simulink model "simulator_prototype_v2"  (R2021b)
settings: Solver=VariableStepAuto  StartTime=0.0  StopTime=60  FixedStep=0.0001  RelTol=1e-4
undefined symbols (not defined in the file or in its folder): X, Y, Z
libraries: sm_lib x47, nesl_utility x7
(part 13 of 13)

== matlab function simulator_prototype_v2/Energy Analysis/MATLAB Function ==
  data: dq input; T output; H input
function T = Kinetic_Energy(dq, H)
T = real((1/2)*transpose(dq)*H*dq);

== matlab function simulator_prototype_v2/Energy Analysis/potential_energy ==
  data: q1 input; U output; q2 input; q3 input; q4 input; q5 input; q6 input
function U = potential_energy(q1,q2,q3,q4,q5,q6)
%#codegen

%    This function was generated by the Symbolic Math Toolbox version 9.0.
%    12-Oct-2021 13:17:17

t2 = conj(q1);
t3 = conj(q2);
t4 = conj(q3);
t5 = conj(q4);
t6 = conj(q5);
t7 = conj(q6);
t24 = 9.007199254740992e+15;
t8 = cos(t2);
t9 = cos(t3);
t10 = cos(t5);
t11 = cos(t6);
t12 = cos(t7);
t13 = sin(t2);
t14 = sin(t3);
t15 = sin(t5);
t16 = sin(t6);
t17 = sin(t7);
t18 = t2+t3;
t26 = (t4.*t24)./9.007199254740992e+15;
t29 = t4.*t24.*1.110223024625157e-16i;
t19 = cos(t18);
t20 = sin(t18);
t27 = cos(t26);
t28 = sin(t26);
t30 = -t29;
t31 = exp(t29);
t21 = t20.*4.602992943936994e+15;
t22 = t19.*7.742227997977903e+15;
t32 = -t27;
t33 = exp(t30);
t34 = t28.*1i;
t38 = t27.*7.38843356682345e-1;
t39 = t27.*2.61156643317655e-1;
t23 = -t21;
t35 = t33-1.0;
t37 = t27+t34;
t40 = t32+t34+1.0;
t42 = t10.*t24.*t28.*(t21-t22).*(-1.232595164407831e-32);
t43 = t15.*t24.*t28.*(t21-t22).*(-1.232595164407831e-32);
t44 = (t10.*t24.*t28.*(t21-t22))./8.112963841460668e+31;
t45 = t38+2.61156643317655e-1;
t46 = t39+7.38843356682345e-1;
t25 = t22+t23;
t36 = t35.^2;
t41 = t40.^2;
t47 = t19.*t45;
t48 = t20.*t46;
t49 = t20.*t37.*t41.*2.196325630278387e-1;
t50 = t19.*t37.*t41.*2.196325630278387e-1;
t51 = -t49;
t52 = -t50;
t53 = t47+t51;
t54 = t48+t52;
t55 = t10.*t54;
t56 = t11.*t53;
t57 = t15.*t54;
t58 = t43+t55;
t59 = t44+t57;
t60 = t16.*t59;
t61 = -t60;
t62 = t56+t61;
et1 = t8.*9.734313376175611e-2-t13.*2.717189118622151e-2;
et2 = t19.*3.161090981652867e-3+t20.*4.486342129859745e-3;
et3 = t47.*1.123016940370151e-2+t48.*9.0769442339979e-4;
et4 = t55.*1.663769266031448e-3+t56.*1.03455776890854e-3;
et5 = t57.*(-1.834077274308e-6)-t60.*1.03455776890854e-3;
et6 = t8.*t9.*1.805586507105727e-2;
et7 = t8.*t14.*2.789883597074818e-2;
et8 = t9.*t13.*2.789883597074818e-2;
et9 = t13.*t14.*(-1.805586507105727e-2);
et10 = t16.*t53.*1.33075164870018e-3+t11.*t59.*1.33075164870018e-3;
et11 = t12.*t58.*7.12549896598485e-4+t12.*t62.*1.31098441441266e-3;
et12 = t17.*t58.*(-1.31098441441266e-3)+t17.*t62.*7.12549896598485e-4;
et13 = t8.*t9.*t27.*7.73459091191916e-3;
et14 = t8.*t14.*t27.*(-4.598452461113469e-3);
et15 = t9.*t13.*t27.*(-4.598452461113469e-3);
et16 = t13.*t14.*t27.*(-7.73459091191916e-3);
et17 = t19.*t31.*t36.*(-1.993592526573721e-4);
et18 = t20.*t31.*t36.*(-1.027576994682181e-3);
et19 = t20.*t37.*t41.*(-1.438933894689597e-3);
et20 = t10.*t24.*t28.*(t21-t22).*(-2.260674779462336e-38);
et21 = t15.*t24.*t28.*(t21-t22).*(-2.050753952000729e-35);
U = real(et1+et2+et3+et4+et5+et6+et7+et8+et9+et10+et11+et12+et13+et14+et15+et16+et17+et18+et19+et20+et21);
